simulink model "PV_test"  (R2016a)
settings: Solver=VariableStepAuto  StartTime=0.0  StopTime=5  RelTol=1e-3
libraries: powerlib x3, re_lib x1
settings Model: Creator=Rangga  LastModifiedBy=Rangga

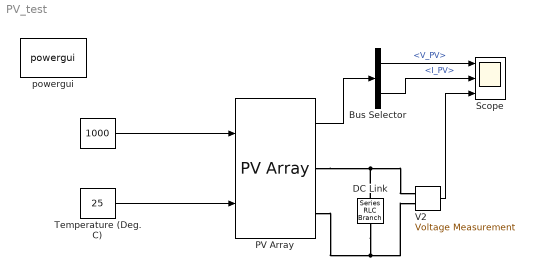
== system PV_test ==
  " " : Constant  Value=1000
  Bus Selector : BusSelector  OutputSignals=V_PV,I_PV
  DC Link : powerlib/Elements/Series RLC Branch  LConnTagsString=__new0  RConnTagsString=__new0  BranchType=C  Resistance=1.0  Inductance=1.0  SetiL0=off  InitialCurrent=0  Capacitance=3000e-6  Setx0=on  InitialVoltage=10  Measurements=None
  PV Array : re_lib/Solar/PV Array  Npar=1  Nser=1  PlotType=one module @ 25 deg.C & specified irradiances  S_vec=1000  Temp_C_vec=[ 45 25 100 ]  ModuleName=User-defined  PlotWhenSelected=off  Pm=99.981  Ncell=36  Voc=22.5  Isc=5.75  Vm=18.9  Im=5.29  beta_Voc_pc=-0.35  alpha_Isc_pc=0.06  beta_Voc=-0.07875  alpha_Isc=0.00345  IL=5.7591  I0=1.3543e-10  nI=0.99573  Rsh=93.7325  Rs=0.14801  BAL=on  Tc=1e-6  Tfilter=5e-5
      settings: AttributesFormatString=|
      | %<ModuleName>
      | %<Nser>-module string
      | %<Npar> parallel strings
  Scope : Scope  NumInputPorts=3
  Temperature (Deg. C) : Constant  Value=25
  V2 : powerlib/Measurements/Voltage Measurement  Tag=PoWeRsYsTeMmEaSuReMeNt  PhasorSimulation=off  OutputType=Magnitude  PSBequivalent=0
  powergui : powerlib/powergui  Priority=1  SimulationMode=Discrete  SolverType=Tustin/Backward Euler (TBE)  SampleTime=50e-6  frequency=60  SPID=off  DisableSnubberDevices=off  DisableRonSwitches=off  DisableVfSwitches=off  SwTol=0  DisplayEquations=off  Interpol=off  ExternalGateDelay=off  methode=off  Ts=10  FunctionMessages=off  echomessages=off  HookPort=off  EnableUseOfTLC=off  x0status=blocks  frequencyindice=0  Pbase=100e6  ErrMax=1e-4  Iterations=50  UnitsV=kV  UnitsW=MW  buscounter=0  RestoreLinks=warning  ResistiveCurrentMeasurement=off  Frange=[0:2:500]  Ylog=off  Xlog=on  ShowGrid=off  save=off  variable=ZData  structure=0  ZoomFFT=off  StartTime=0.0  cycles=1  DisplayStyle=1  fundamental=60  FreqAxis=off  MaxFrequency=1000  frequencyindicesteady=1  RmsSteady=1  display=off
  wires:
  " "/1 -> PV Array/1
  Temperature (Deg. C)/1 -> PV Array/2
  PV Array/1 -> Bus Selector/1
  Bus Selector/1 -> Scope/1  "<V_PV>"
  Bus Selector/2 -> Scope/2  "<I_PV>"
  V2/1 -> Scope/3
  connections:
  PV Array/RConn1 -- DC Link/LConn1 -- V2/LConn1
  PV Array/RConn2 -- DC Link/RConn1 -- V2/LConn2
